simulink model "single_model_test"  (R2024a)
settings: Solver=VariableStepAuto  StartTime=0.0  StopTime=inf  RelTol=1e-3
undefined symbols (not defined in the file): f
libraries: instrumentlib x1
settings Model: Creator=thecez  LastModifiedBy=thecez

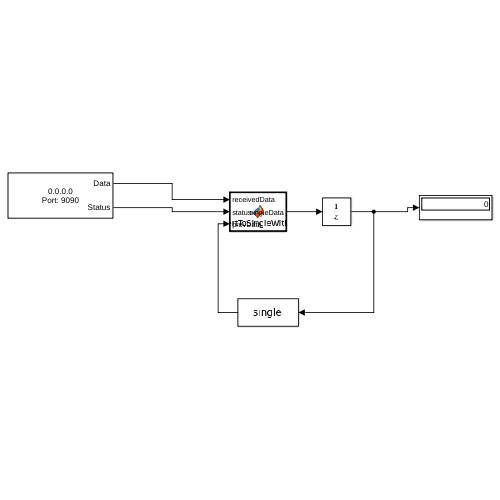
[thumbnail: Simulink's stored preview of the top-level diagram]
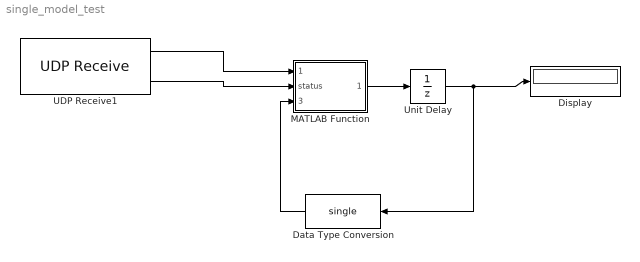
== system single_model_test ==
  Data Type Conversion : DataTypeConversion  OutMin=[1]  OutMax=[1]  OutDataTypeStr=single  SaturateOnIntegerOverflow=off  RndMeth=Floor
  Display : Display
      settings: Format=decimal (Stored Integer)
  MATLAB Function : MATLAB Function  TreatAsAtomicUnit=on
  UDP Receive1 : instrumentlib/UDP Receive  LocalAddress=0.0.0.0  LocalPort=9090  EnablePortSharing=off  Host=localhost  Port=9090  GetLatestData=off  DataSize=[ 1, 1 ]  DataType=single  ASCIIFormatting=%f,  Terminator=LF  CustomTerminator=10  ByteOrder=big-endian  EnableBlockingMode=off  Timeout=10  SampleTime=0.01  SimulateUsing=Interpreted execution
  Unit Delay : UnitDelay  InitialCondition=single(0)  SampleTime=-1  HasFrameUpgradeWarning=on
  wires:
  MATLAB Function/1(singleData) -> Unit Delay/1
  UDP Receive1/2 -> MATLAB Function/2(status)
  Data Type Conversion/1 -> MATLAB Function/3(prevData)
  Unit Delay/1 -> Data Type Conversion/1, Display/1
  UDP Receive1/1 -> MATLAB Function/1(receivedData)

== matlab function single_model_test/MATLAB Function ==
  data: receivedData input; singleData output; status input; prevData input
function singleData = convertToSingleWithHold(receivedData, status, prevData)
    % Convert received data to single precision and retain previous value if no new data
    %
    % Inputs:
    %   receivedData - Input data (e.g., double, uint8, etc.)
    %   status       - Status flag (1 = process data, 0 = hold previous value)
    %   prevData     - Previous output value (fed back into the function)
    %
    % Outputs:
    %   singleData   - Data converted to single precision or retained previous value

    persistent rows cols currentRow currentCol matrix;

    % Check if prevData is empty (first iteration)
    if isempty(prevData)
        % Initialize singleData with a default value
        singleData = single(0); % Default initialization
        return;
    end

    % Initialize persistent variables
    if isempty(rows) || (single(receivedData) == -1  && status == 1)
        rows = single(-1);          % Initialize rows as -1
        cols = single(-1);          % Initialize cols as -1
        currentRow = 1;     % Start filling from the first row
        currentCol = 1;     % Start filling from the first column
        matrix = zeros(500, 500);        % Initialize matrix as empty
        singleData = single(0);
        return
    end

    

    if status == 1
        if rows == -1
            % If rows are not set, set rows from received data
            rows = typecast(receivedData, 'single');  % Decode float32 value for rows
            singleData = single(receivedData);
            return;
        elseif cols == -1
            % If cols are not set, set cols from received data
            cols = typecast(receivedData, 'single');  % Decode float32 value for cols
            matrix = zeros(rows, cols);              % Preallocate matrix after dimensions are known
            singleData = single(receivedData);
            return;
        else
            % Process incoming data and fill the matrix row by row, column by column
            singleData = typecast(receivedData, 'single');  % Decode float32 value
            
            if currentRow <= rows && currentCol <= cols
                matrix(currentRow, currentCol) = singleData;  % Fill the current cell in the matrix
                
                % Move to the next column or row when a row is complete
                currentCol = currentCol + 1;
                if currentCol > cols
                    currentCol = 1;          % Reset column index to 1
                    currentRow = currentRow + 1;  % Move to the next row
                    
                    if currentRow > rows
                        disp("Matrix reconstruction complete!");
                        disp(matrix);       % Display the reconstructed matrix in Command Window

                        % Reset persistent variables for the next cycle
                        rows = single(-1);
                        cols = single(-1);
                        currentRow = 1;
                        currentCol = 1;
                        singleData = single(0);  % Reset output to default value
                        return;
                    end
                end
            end
        end
    else
        % If no new data, retain the previous value
        singleData = single(prevData);
    end

end
